simulink model "chap9_7sim"  (Simulink 5.0)
settings: Solver=ode45  StartTime=0.0  StopTime=10  RelTol=1e-3
settings Model: LastModifiedBy=Administrator

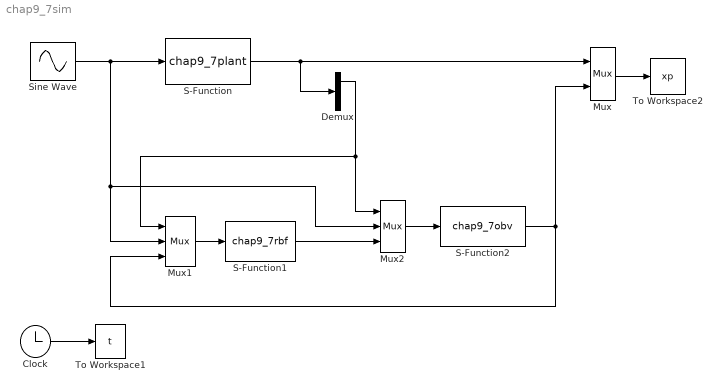
== system chap9_7sim ==
  Clock : Clock
      settings: Decimation=10
  Demux : Demux  Outputs=2
  Mux : Mux  Inputs=2
  Mux1 : Mux  Inputs=3
  Mux2 : Mux  Inputs=3
  S-Function : S-Function  FunctionName=chap9_7plant
  S-Function1 : S-Function  FunctionName=chap9_7rbf
  S-Function2 : S-Function  FunctionName=chap9_7obv
  Sine Wave : Sin  SampleTime=0
  To Workspace1 : ToWorkspace  VariableName=t  SampleTime=-1  SaveFormat=Array
  To Workspace2 : ToWorkspace  VariableName=xp  SampleTime=-1  SaveFormat=Array
  wires:
  Sine Wave/1 -> S-Function/1, Mux2/2, Mux1/2
  Clock/1 -> To Workspace1/1
  Mux/1 -> To Workspace2/1
  S-Function2/1 -> Mux/2, Mux1/3
  Mux1/1 -> S-Function1/1
  Mux2/1 -> S-Function2/1
  S-Function1/1 -> Mux2/3
  S-Function/1 -> Mux/1, Demux/1
  Demux/1 -> Mux2/1, Mux1/1
